simulink model "flight_simulator"  (R2021a)
settings: Solver=VariableStepAuto  StartTime=0.0  StopTime=1000.0  RelTol=1e-3
libraries: aerolibfltsims x2, AE512Blockset x2
settings Model: Creator=maxab  LastModifiedBy=maxab

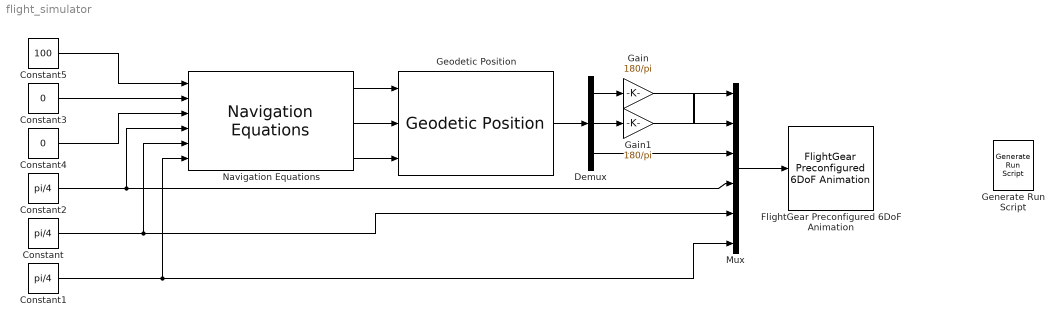
== system flight_simulator ==
  Constant : Constant  Value=pi/4
  Constant1 : Constant  Value=pi/4
  Constant2 : Constant  Value=pi/4
  Constant3 : Constant  Value=0
  Constant4 : Constant  Value=0
  Constant5 : Constant  Value=100
  Demux : Demux  Outputs=3
  FlightGear Preconfigured 6DoF Animation : aerolibfltsims/FlightGear Preconfigured 6DoF Animation  xFlightGearVersion=v2019.1  DestinationIpAddress=127.0.0.1  DestinationPort=5502  SampleTime=1/30  packetVersion=24
  Gain : Gain  Gain=180/pi
  Gain1 : Gain  Gain=180/pi
  Generate Run Script : aerolibfltsims/Generate Run Script  Architecture=Win64  dataFlow=Send  GeometryModelName=c172p  AirportId=PHNL  RunwayId=08L  InitialAltitude=7224  InitialHeading=113  OffsetDistance=4.72  OffsetAzimuth=0  InstallScenery=off  DisableShaders=on  OriginAddress=127.0.0.1  DestinationPort=5502  OriginPort=5505  LocalAddress=127.0.0.1  OutputFileName=runfg.bat  FlightGearBaseDirectory=C:\Program Files\FlightGear 2020.3
  Geodetic Position : AE512Blockset/Geodetic Position  Xgeodetic0=Xgeodetic0
  Mux : Mux  Inputs=6
  Navigation Equations : AE512Blockset/Navigation Equations  Description=|
      | Version History  
      |                  
      | 05/24/05: Created
  wires:
  Mux/1 -> FlightGear Preconfigured 6DoF Animation/1
  Constant1/1 -> Navigation Equations/6, Mux/6
  Constant/1 -> Mux/5, Navigation Equations/5
  Constant2/1 -> Navigation Equations/4, Mux/4
  Navigation Equations/1 -> Geodetic Position/1
  Navigation Equations/2 -> Geodetic Position/2
  Navigation Equations/3 -> Geodetic Position/3
  Geodetic Position/1 -> Demux/1
  Demux/1 -> Gain/1
  Demux/2 -> Gain1/1
  Gain1/1 -> Mux/1
  Gain/1 -> Mux/2
  Demux/3 -> Mux/3
  Constant5/1 -> Navigation Equations/1
  Constant3/1 -> Navigation Equations/2
  Constant4/1 -> Navigation Equations/3
